simulink model "pendulum"  (R2024b)
settings: Solver=VariableStepAuto  StartTime=0.0  StopTime=10.0  RelTol=1e-3
values from neighbouring files (symbols this model uses):
  b = 0.5    [pendulum_initail_value.m]
  F = 0    [pendulum_initail_value.m]
  g = 9.81    [pendulum_initail_value.m]
  J = m*l1^2    (= 1.35)    [pendulum_initail_value.m]
  l1 = 1    [pendulum_initail_value.m]
  m = 1.35    [pendulum_initail_value.m]
settings Model: Creator=Aluno  LastModifiedBy=Aluno

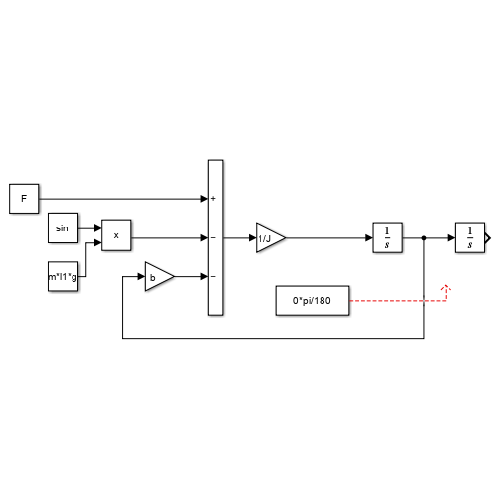
[thumbnail: Simulink's stored preview of the top-level diagram]
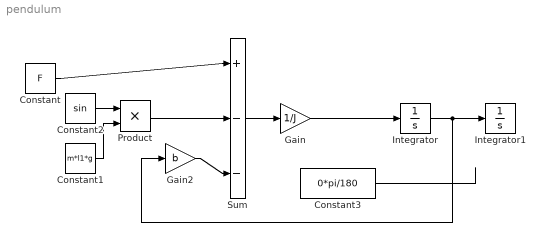
== system pendulum ==
  Constant : Constant  Value=F
  Constant1 : Constant  Value=m*l1*g
  Constant2 : Constant  Value=sin
  Constant3 : Constant  Value=0*pi/180
  Gain : Gain  Gain=1/J
  Gain2 : Gain  Gain=b
  Integrator : Integrator
  Integrator1 : Integrator
  Product : Product
  Sum : Sum  Inputs=|+|-|-|
  wires:
  Constant/1 -> Sum/1
  Product/1 -> Sum/2
  Constant1/1 -> Product/2
  Constant2/1 -> Product/1
  Sum/1 -> Gain/1
  Gain2/1 -> Sum/3
  Gain/1 -> Integrator/1
  Integrator/1 -> Gain2/1, Integrator1/1
  Constant3/1 -> ?
